simulink model "gamma"  (R2021a)
settings: Solver=VariableStepAuto  StartTime=0.0  StopTime=inf  RelTol=1e-3
libraries: robotlib x3
settings Model: Creator=julio  LastModifiedBy=julio

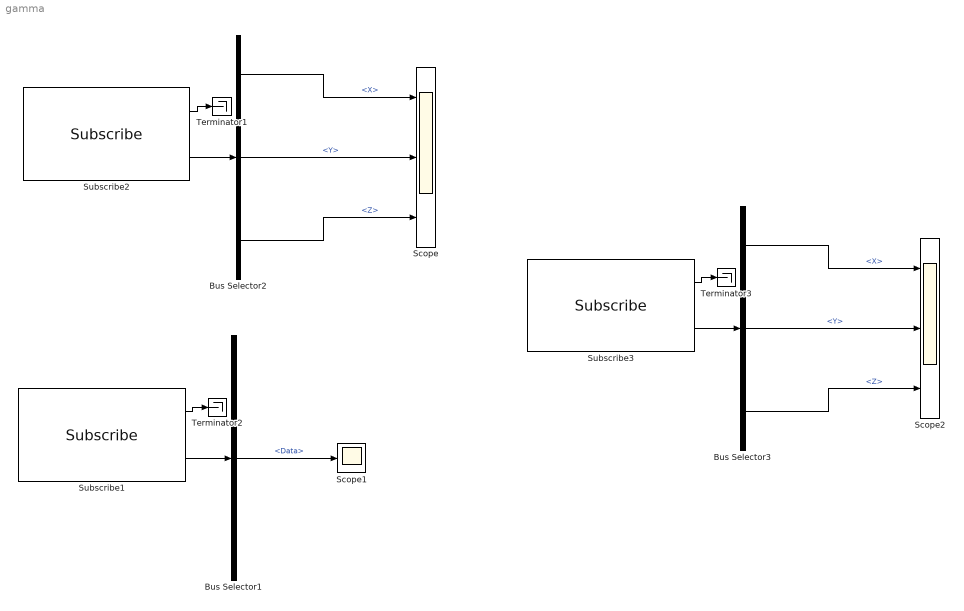
== system gamma ==
  Bus Selector1 : BusSelector  OutputSignals=Data
  Bus Selector2 : BusSelector  OutputSignals=Linear.X,Linear.Y,Linear.Z
  Bus Selector3 : BusSelector  OutputSignals=Linear.X,Linear.Y,Linear.Z
  Scope : Scope  NumInputPorts=3
  Scope1 : Scope
  Scope2 : Scope  NumInputPorts=3
  Subscribe1 : robotlib/Subscribe  topicSource=Select from ROS network  topic=/crazyflie/leader_u  messageType=std_msgs/Float32  SampleTime=-1  legacyBusStruct=off  messageQueueLength=1
  Subscribe2 : robotlib/Subscribe  topicSource=Select from ROS network  topic=/crazyflie/cmd_vel  messageType=geometry_msgs/Twist  SampleTime=-1  legacyBusStruct=off  messageQueueLength=1
  Subscribe3 : robotlib/Subscribe  topicSource=Select from ROS network  topic=/crazyflie/gamma  messageType=geometry_msgs/Twist  SampleTime=-1  legacyBusStruct=off  messageQueueLength=1
  Terminator1 : Terminator
  Terminator2 : Terminator
  Terminator3 : Terminator
  wires:
  Bus Selector2/3 -> Scope/3  "<Z>"
  Subscribe2/2 -> Bus Selector2/1
  Bus Selector2/2 -> Scope/2  "<Y>"
  Subscribe2/1 -> Terminator1/1
  Bus Selector2/1 -> Scope/1  "<X>"
  Subscribe1/1 -> Terminator2/1
  Subscribe1/2 -> Bus Selector1/1
  Bus Selector1/1 -> Scope1/1  "<Data>"
  Subscribe3/1 -> Terminator3/1
  Bus Selector3/3 -> Scope2/3  "<Z>"
  Subscribe3/2 -> Bus Selector3/1
  Bus Selector3/1 -> Scope2/1  "<X>"
  Bus Selector3/2 -> Scope2/2  "<Y>"
